simulink model "dobdesign"  (R2022b)
settings: Solver=FixedStepAuto  StartTime=0.0  StopTime=inf  FixedStep=0.02  RelTol=1e-3
values from neighbouring files (symbols this model uses):
  acri = atan(1/theta)    [transfer.m]
  Cfa = 15000    [transfer.m]
  D = 0    [transfer.m]
  Fz = (m*g)/4    (= 3801.375)    [transfer.m]
  J = 2392    [transfer.m]
  m = 1550    [transfer.m]
  mu = 1    [transfer.m]
  V = 30    [transfer.m]
libraries: cstblocks x4, simulink x2, simulink_extras x1, fuzblock x1, slpidlib x1, vehdynlibviscommon x1
settings Model: Creator=clkgo  LastModifiedBy=clkgo
settings SolverCC: AlgebraicLoopSolver=TrustRegion
settings DebuggingCC: UnconnectedInputMsg=warning  UnconnectedOutputMsg=warning  UnconnectedLineMsg=warning  SFMachineParentedDataDiag=warning
settings ModelReferenceCC: EnableRefExpFcnMdlSchedulingChecks=on
settings RTWCC: DLArmComputeVersion=19.05

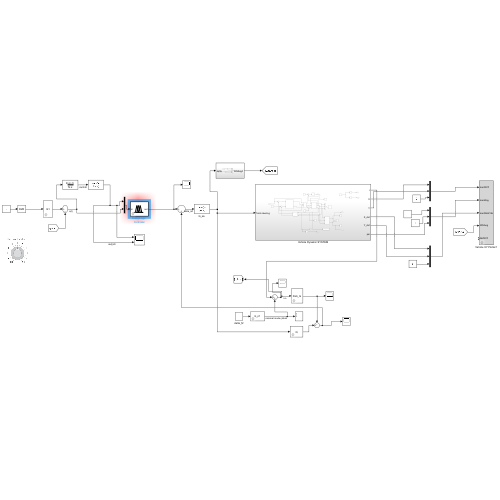
[thumbnail: Simulink's stored preview of the top-level diagram]
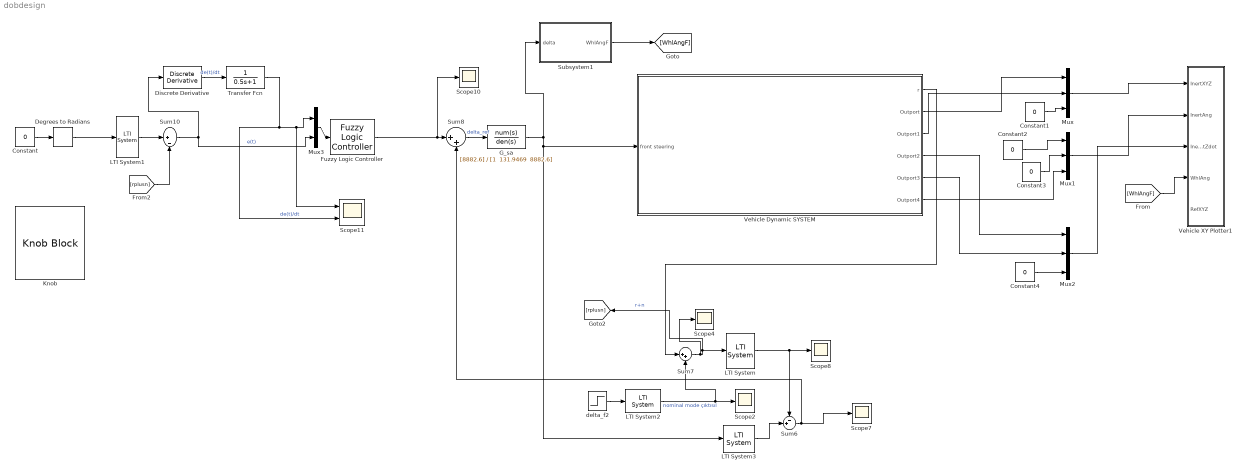
== system dobdesign ==
  Constant{,1..4} (5 alike) : Constant  Value=0
  Degrees to Radians : simulink_extras/Transformations/Degrees to Radians
  Discrete Derivative : simulink/Discrete/Discrete Derivative  gainval=1.0  ICPrevScaledInput=0.0  OutMin=[]  OutMax=[]  OutDataType=fixdt(1, 16)  OutScaling=2^-10  DoSatur=off
  Fuzzy Logic Controller : fuzblock/Fuzzy Logic  Controller  FIS=dobfuzzy14  OutputSampleNumber=101  DataType=double  FuzzifiedInputs=off  RuleFiringStrengths=off  RuleOutputs=off  AggregatedOutputs=off  SimulateUsing=Interpreted execution  OutOfRangeInputValueMessage=warning  NoRuleFiredMessage=warning  EmptyOutputFuzzySetMessage=warning
  "G_sa " : TransferFcn  Numerator=[8882.6]  Denominator="[1  131.9469  8882.6]"
  Knob : KnobBlock  ScaleMin=-10  ScaleMax=10
  LTI System : cstblocks/LTI System  sys=Dob_G  IC=[]
  LTI System1 : cstblocks/LTI System  sys=G1  IC=[]
  LTI System2 : cstblocks/LTI System  sys=G_n1  IC=[]
  LTI System3 : cstblocks/LTI System  sys=Q  IC=[]
  Mux : Mux  Inputs=3
  Mux1 : Mux  Inputs=3
  Mux2 : Mux  Inputs=3
  Mux3 : Mux  Inputs=2
  Scope{2,4,7..8,10} (5 alike) : Scope
  Scope11 : Scope  NumInputPorts=2
  Subsystem1 : Subsystem
  Sum10 : Sum  Inputs=|+-
  Sum6 : Sum  Inputs=-+|
  Sum7 : Sum  Inputs=|++
  Sum8 : Sum  Inputs=|++
  Transfer Fcn : TransferFcn  Denominator=[0.5 1]
  Vehicle Dynamic SYSTEM : Subsystem
  Vehicle XY Plotter1 : Subsystem  mask(Vehicle XY Plotter){extRef=on, extStats=off, extTireF=off, a=2, b=2, w=2, figBorder=10, bufferSize=1024, velNorm=5, tireFNorm=1000, pltDT=0.2}
      mask prompts: extRef "Plot path reference, extRef"; extStats "Display speed, RPM and Gear"; extTireF "Display tire forces"; a "Distance to front axle from CG, a [m]:"; b "Distance to rear axle from CG, b [m]:"; w "Track width, w [m]:"; figBorder "Distance to figure borders, figBorder [m]:"; bufferSize "Path buffer sampe size, bufferSize []:"; velNorm "Velocity vector scaling, velNorm [m*s/m]:"; tireFNorm "Tire force vector scaling, tireFNorm [m/N]:"; pltDT "Plot update rate, pltDT [s]:"
      mask help:
      | This block will display a MATLAB figure which indicates the vehicle path, current position and heading velocity.
      | An optional path reference is also provided.
      mask init:
      | block = gcb;
      | if autoblkschecksimstopped(block)
      |     ParamNames = {'extRef';'extStats';'extTireF';'extTireF'};
      |     PortNames = {'RefXYZ';'Stats';'TireFx';'TireFy'};
      |     for idx=1:length(PortNames)
      |         InportOption  = {'built-in/Ground', [PortNames{idx}, ' Ground'];...
      |             'built-in/Inport',PortNames{idx}};
      |         if ~strcmp(get_param(block,ParamNames{idx}),'on')
      |             NewBlkHdl = autoblksreplaceblock(block, InportOption, 1);
      |             set_param(NewBlkHdl, 'ShowName', 'off');
      |         else
      |             autoblksreplaceblock(block, InportOption, 2);
      |         end
      |     end
      |     InportNames = {'InertXYZ';'InertAng';'InertXdotYdotZdot';'WhlAng';'RefXYZ';'Stats';'TireFx';'TireFy'};
      |     FoundNames = get_param(find_system(block, 'LookUnderMasks', 'all', 'SearchDepth', 1, 'FollowLinks', 'on', 'BlockType', 'Inport'), 'Name');
      |     [~,PortI] = intersect(InportNames, FoundNames);
      |     PortI = sort(PortI);
      |     for idx = 1:length(PortI)
      |         set_param([block, '/', InportNames{PortI(idx)}], 'Port', num2str(idx));
      |     end
      | end
      mask TypeOptions a: Vehicle XY Plotter/a
      mask TypeOptions b: Vehicle XY Plotter/b
      mask TypeOptions w: Vehicle XY Plotter/w
      mask TypeOptions figBorder: Vehicle XY Plotter/figBorder
      mask TypeOptions bufferSize: Vehicle XY Plotter/bufferSize
      mask TypeOptions velNorm: Vehicle XY Plotter/velNorm
      mask TypeOptions tireFNorm: Vehicle XY Plotter/tireFNorm
      mask DialogControl Container3 Prompt: Plot and Display Options
  delta_f2 : Step  Time=0.1  After=0  SampleTime=0
  wires:
  Vehicle Dynamic SYSTEM/1(r) -> Sum7/1
  LTI System/1 -> Sum6/1, Scope8/1
  LTI System2/1 -> Scope2/1, Sum7/2  "nominal mode çıktısıl"
  "G_sa "/1 -> LTI System3/1, Vehicle Dynamic SYSTEM/1(front steering), Subsystem1/1(delta)
  Sum7/1 -> Scope4/1, LTI System/1, [rplusn]  "r+n"
  LTI System3/1 -> Sum6/2
  Sum6/1 -> Sum8/2, Scope7/1
  Sum8/1 -> "G_sa "/1  "delta_ref"
  delta_f2/1 -> LTI System2/1
  [rplusn] -> Sum10/2
  LTI System1/1 -> Sum10/1
  Degrees to Radians/1 -> LTI System1/1
  Sum10/1 -> Mux3/2, Discrete Derivative/1  "e(t)"
  Mux3/1 -> Fuzzy Logic Controller/1
  Discrete Derivative/1 -> Transfer Fcn/1  "de(t)/dt"
  Transfer Fcn/1 -> Scope11/2, Scope11/1, Mux3/1  "de(t)/dt"
  Fuzzy Logic Controller/1 -> Scope10/1, Sum8/1
  Constant/1 -> Degrees to Radians/1
  Subsystem1/1(WhlAngF) -> [WhlAngF]
  Vehicle Dynamic SYSTEM/2(Outport) -> Mux/1
  Vehicle Dynamic SYSTEM/3(Outport1) -> Mux/2
  Constant1/1 -> Mux/3
  Mux/1 -> Vehicle XY Plotter1/1(InertXYZ)
  Constant2/1 -> Mux1/1
  Constant3/1 -> Mux1/2
  Vehicle Dynamic SYSTEM/6(Outport4) -> Mux1/3
  Mux1/1 -> Vehicle XY Plotter1/2(InertAng)
  Vehicle Dynamic SYSTEM/4(Outport2) -> Mux2/1
  Vehicle Dynamic SYSTEM/5(Outport3) -> Mux2/2
  Constant4/1 -> Mux2/3
  Mux2/1 -> Vehicle XY Plotter1/3(InertXdotYdotZdot)
  [WhlAngF] -> Vehicle XY Plotter1/4(WhlAng)

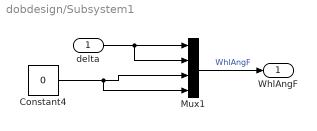
== system dobdesign/Subsystem1 ==
  delta : Inport
  Constant4 : Constant  Value=0
  Mux1 : Mux
  WhlAngF : Outport
  wires:
  delta/1 -> Mux1/2, Mux1/1
  Mux1/1 -> WhlAngF/1  "WhlAngF"
  Constant4/1 -> Mux1/4, Mux1/3

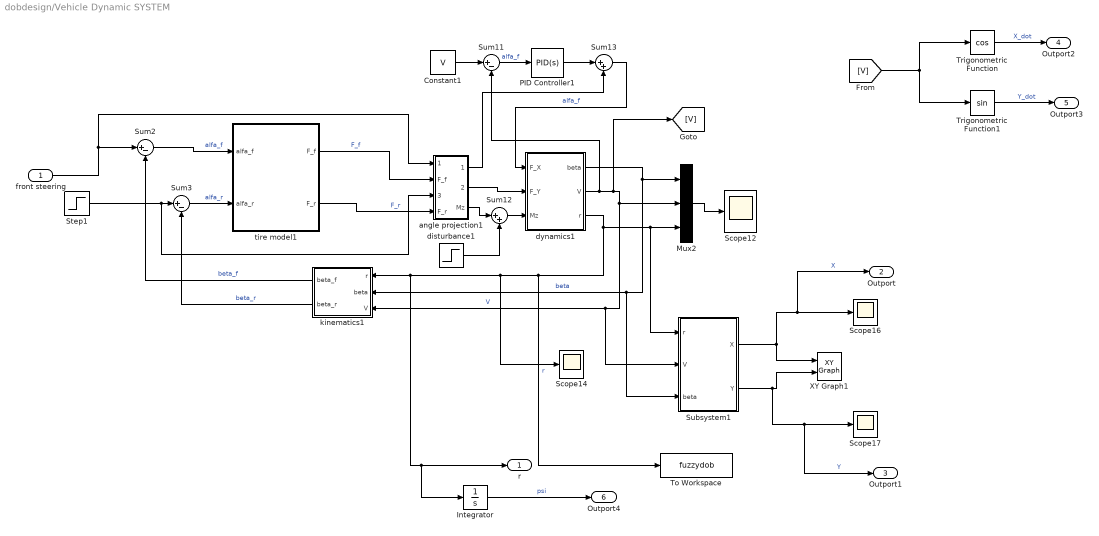
== system dobdesign/Vehicle Dynamic SYSTEM ==
  front steering : Inport
  Constant1 : Constant  Value=V
  Integrator : Integrator
  Mux2 : Mux  Inputs=3
  PID Controller1 : slpidlib/PID Controller  Controller=PID  Form=Parallel  TimeDomain=Continuous-time  UseExternalTs=off  SampleTime=-1  IntegratorMethod=Forward Euler  FilterMethod=Forward Euler  ControllerParametersSource=internal  P=60000  I=1000  D=0  UseFilter=on  N=100  TunerSelectOption=Transfer Function Based (PID Tuner App)  InitialConditionSource=internal  InitialConditionForIntegrator=0  InitialConditionForFilter=0  DifferentiatorICPrevScaledInput=0  ExternalReset=none  TrackingMode=off  Kt=1  LimitOutput=off  SatLimitsSource=internal  UpperSaturationLimit=inf  LowerSaturationLimit=-inf  LinearizeAsGain=on  AntiWindupMode=none  Kb=1  POutMin=[]  POutMax=[]  IOutMin=[]  IOutMax=[]  DOutMin=[]  DOutMax=[]  NOutMin=[]  NOutMax=[]  SumOutMin=[]  SumOutMax=[]  SaturationOutMin=[]  SaturationOutMax=[]  PParamMin=[]  PParamMax=[]  IParamMin=[]  IParamMax=[]  DParamMin=[]  DParamMax=[]  NParamMin=[]  NParamMax=[]  KbParamMin=[]  KbParamMax=[]  KtParamMin=[]  KtParamMax=[]  KbOutMin=[]  KbOutMax=[]  KtOutMin=[]  KtOutMax=[]  IntegratorOutMin=[]  IntegratorOutMax=[]  FilterOutMin=[]  FilterOutMax=[]  SumI1OutMin=[]  SumI1OutMax=[]  SumI2OutMin=[]  SumI2OutMax=[]  SumI3OutMin=[]  SumI3OutMax=[]  SumI4OutMin=[]  SumI4OutMax=[]  SumDOutMin=[]  SumDOutMax=[]  DifferentiatorOutMin=[]  DifferentiatorOutMax=[]  FilterDiffOutCoefMin=[]  FilterDiffOutCoefMax=[]  ReciprocalOutMin=[]  ReciprocalOutMax=[]  SumDenOutMin=[]  SumDenOutMax=[]  SumNumOutMin=[]  SumNumOutMax=[]  DivideOutMin=[]  DivideOutMax=[]  UdiffTsProdOutMin=[]  UdiffTsProdOutMax=[]  NTsProdOutMin=[]  NTsProdOutMax=[]  UintegralTsProdOutMin=[]  UintegralTsProdOutMax=[]  UngainTsProdOutMin=[]  UngainTsProdOutMax=[]  IntegratorContinuousStateAttributes=''  IntegratorStateMustResolveToSignalObject=off  IntegratorRTWStateStorageClass=Auto  FilterContinuousStateAttributes=''  FilterStateMustResolveToSignalObject=off  FilterRTWStateStorageClass=Auto  ParallelPVariant=InternalParameters  IdealPVariant=Disabled  IVariant=InternalParameters  DVariant=InternalParameters  IntegratorVariant=Continuous  SatVariant=Disabled  AWVariant=Passthrough  PCopyVariant=Disabled  TRVariant=Disabled  FdbkBlocksVariant=Forward  IdealPFdbkVariant=Disabled  SatFdbkVariant=Disabled  DerivativeFilterVariant=ContFilter  NVariant=InternalParameters  NCopyVariant=Disabled  FilterICVariant=InternalICsFilter  IntegratorICVariant=InternalICs  ExternalResetVariant=Disabled  TRSumVariant=Passthrough  SumFdbkVariant=Disabled  SumVariant=Sum_PID  TsampFilterVariant=InternalTs  TsampNgainVariant=Passthrough  TsampIntegralVariant=Passthrough  ExternalSaturationOutDataTypeStr=Inherit: Same as second input
  Scope{12,14,16..17} (4 alike) : Scope
  Step1 : Step  Time=0.1  After=0  SampleTime=0
  Subsystem1 : Subsystem
  Sum11 : Sum  Inputs=|+-
  Sum12 : Sum  Inputs=|++
  Sum13 : Sum  Inputs=|++
  Sum2 : Sum  Inputs=|+-
  Sum3 : Sum  Inputs=|+-
  To Workspace : ToWorkspace  VariableName=fuzzydob  SaveFormat=Timeseries  SampleTime=-1
  Trigonometric Function : Trigonometry  Operator=cos
  Trigonometric Function1 : Trigonometry
  XY Graph1 : simulink/Sinks/XY Graph  xmin=0  xmax=500  ymin=0  ymax=50  st=-1
  angle projection1 : Subsystem
  disturbance1 : Step  Time=2  After=1000  SampleTime=0
  dynamics1 : Subsystem
  kinematics1 : Subsystem
  tire model1 : Subsystem
  r : Outport
  Outport : Outport  Port=2
  Outport1 : Outport  Port=3
  Outport2 : Outport  Port=4
  Outport3 : Outport  Port=5
  Outport4 : Outport  Port=6
  wires:
  kinematics1/1(beta_f) -> Sum2/2  "beta_f"
  dynamics1/3(r) -> To Workspace/1, Scope14/1, Integrator/1, r/1, kinematics1/1(r), Subsystem1/1(r), Mux2/3  "r"
  Sum2/1 -> tire model1/1(alfa_f)  "alfa_f"
  dynamics1/2(V) -> [V], Subsystem1/2(V), kinematics1/3(V), Mux2/2, Sum11/2  "V"
  dynamics1/1(beta) -> Subsystem1/3(beta), kinematics1/2(beta), Mux2/1  "beta"
  kinematics1/2(beta_r) -> Sum3/2  "beta_r"
  Subsystem1/2(Y) -> Outport1/1, Scope17/1, XY Graph1/2  "Y"
  disturbance1/1 -> Sum12/2
  Sum3/1 -> tire model1/2(alfa_r)  "alfa_r"
  PID Controller1/1 -> Sum13/1
  Step1/1 -> angle projection1/3(In3), Sum3/1
  Constant1/1 -> Sum11/1
  tire model1/1(F_f) -> angle projection1/2(F_f)  "F_f"
  angle projection1/3(Mz) -> Sum12/1
  tire model1/2(F_r) -> angle projection1/4(F_r)  "F_r"
  angle projection1/2(F_Y) -> dynamics1/2(F_Y)
  angle projection1/1(F_X) -> Sum13/2
  Mux2/1 -> Scope12/1
  Sum11/1 -> PID Controller1/1  "alfa_f"
  Sum12/1 -> dynamics1/3(Mz)
  front steering/1 -> angle projection1/1(In1), Sum2/1
  Subsystem1/1(X) -> XY Graph1/1, Outport/1, Scope16/1  "X"
  Sum13/1 -> dynamics1/1(F_X)  "alfa_f"
  [V] -> Trigonometric Function/1, Trigonometric Function1/1
  Trigonometric Function/1 -> Outport2/1  "X_dot"
  Trigonometric Function1/1 -> Outport3/1  "Y_dot"
  Integrator/1 -> Outport4/1  "psi"

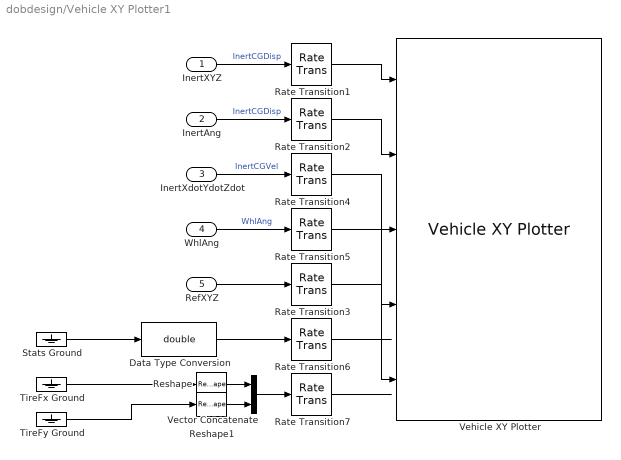
== system dobdesign/Vehicle XY Plotter1 ==
  InertXYZ : Inport
  InertAng : Inport  Port=2
  InertXdotYdotZdot : Inport  Port=3
  WhlAng : Inport  Port=4
  RefXYZ : Inport  Port=5
  Data Type Conversion : DataTypeConversion  OutDataTypeStr=double  SaturateOnIntegerOverflow=off  RndMeth=Floor
  Rate Transition{1..7} (7 alike) : RateTransition  Deterministic=off  OutPortSampleTime=pltDT
  Reshape : Reshape  OutputDimensionality=Row vector (2-D)
  Reshape1 : Reshape  OutputDimensionality=Row vector (2-D)
  Stats Ground : Ground
  TireFx Ground : Ground
  TireFy Ground : Ground
  Vector Concatenate : Concatenate  Mode=Multidimensional array
  Vehicle XY Plotter : vehdynlibviscommon/Vehicle XY Plotter  w=w  a=a  b=b  figBorder=figBorder  bufferSize=bufferSize  extStats=off  extTireF=off
  wires:
  Vector Concatenate/1 -> Rate Transition7/1
  Reshape1/1 -> Vector Concatenate/2
  Reshape/1 -> Vector Concatenate/1
  RefXYZ/1 -> Rate Transition3/1
  Rate Transition7/1 -> ?
  Data Type Conversion/1 -> Rate Transition6/1
  Rate Transition6/1 -> ?
  Rate Transition5/1 -> Vehicle XY Plotter/4
  Rate Transition4/1 -> Vehicle XY Plotter/3
  Rate Transition2/1 -> Vehicle XY Plotter/2
  Rate Transition1/1 -> Vehicle XY Plotter/1
  Rate Transition3/1 -> Vehicle XY Plotter/5
  WhlAng/1 -> Rate Transition5/1  "WhlAng"
  InertXYZ/1 -> Rate Transition1/1  "InertCGDisp"
  InertXdotYdotZdot/1 -> Rate Transition4/1  "InertCGVel"
  InertAng/1 -> Rate Transition2/1  "InertCGDisp"
  Stats Ground/1 -> Data Type Conversion/1
  TireFx Ground/1 -> Reshape/1
  TireFy Ground/1 -> Reshape1/1

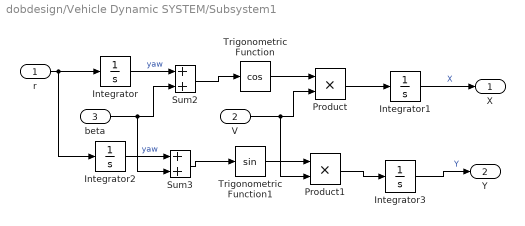
== system dobdesign/Vehicle Dynamic SYSTEM/Subsystem1 ==
  r : Inport
  V : Inport  Port=2
  beta : Inport  Port=3
  Integrator : Integrator
  Integrator1 : Integrator  UpperSaturationLimit=80  LowerSaturationLimit=0
  Integrator2 : Integrator
  Integrator3 : Integrator  UpperSaturationLimit=80  LowerSaturationLimit=0
  Product : Product
  Product1 : Product
  Sum2 : Sum
  Sum3 : Sum
  Trigonometric Function : Trigonometry  Operator=cos
  Trigonometric Function1 : Trigonometry
  X : Outport
  Y : Outport  Port=2
  wires:
  Integrator/1 -> Sum2/1  "yaw"
  V/1 -> Product1/2, Product/2
  Sum2/1 -> Trigonometric Function/1
  Product1/1 -> Integrator3/1
  Trigonometric Function/1 -> Product/1
  Trigonometric Function1/1 -> Product1/1
  Sum3/1 -> Trigonometric Function1/1
  Product/1 -> Integrator1/1
  Integrator2/1 -> Sum3/1  "yaw"
  Integrator3/1 -> Y/1  "Y"
  Integrator1/1 -> X/1  "X"
  beta/1 -> Sum3/2, Sum2/2
  r/1 -> Integrator2/1, Integrator/1

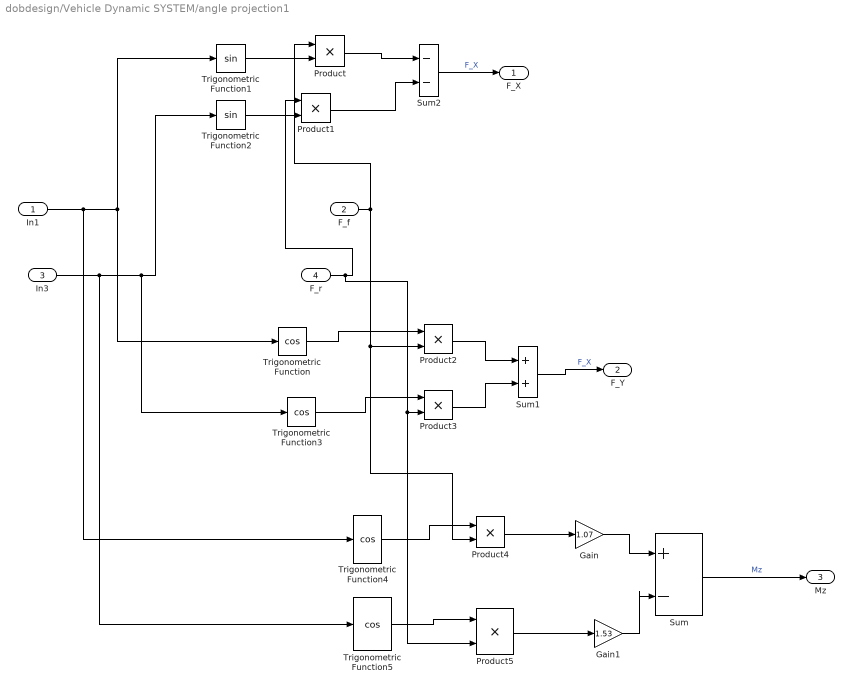
== system dobdesign/Vehicle Dynamic SYSTEM/angle projection1 ==
  In1 : Inport
  F_f : Inport  Port=2
  In3 : Inport  Port=3
  F_r : Inport  Port=4
  Gain : Gain  Gain=1.07
  Gain1 : Gain  Gain=1.53
  Product{,1..5} (6 alike) : Product
  Sum : Sum  Inputs=+-
  Sum1 : Sum
  Sum2 : Sum  Inputs=--
  Trigonometric Function{,3..5} (4 alike) : Trigonometry  Operator=cos
  Trigonometric Function1 : Trigonometry
  Trigonometric Function2 : Trigonometry
  F_X : Outport
  F_Y : Outport  Port=2
  Mz : Outport  Port=3
  wires:
  Trigonometric Function2/1 -> Product1/2
  Sum2/1 -> F_X/1  "F_X"
  Product1/1 -> Sum2/2
  F_f/1 -> Product/1, Product2/2, Product4/2
  Trigonometric Function1/1 -> Product/2
  F_r/1 -> Product5/2, Product3/2, Product1/1
  In3/1 -> Trigonometric Function5/1, Trigonometric Function3/1, Trigonometric Function2/1
  Product/1 -> Sum2/1
  In1/1 -> Trigonometric Function4/1, Trigonometric Function1/1, Trigonometric Function/1
  Trigonometric Function/1 -> Product2/1
  Trigonometric Function3/1 -> Product3/1
  Product2/1 -> Sum1/1
  Product3/1 -> Sum1/2
  Sum1/1 -> F_Y/1  "F_X"
  Trigonometric Function4/1 -> Product4/1
  Trigonometric Function5/1 -> Product5/1
  Product4/1 -> Gain/1
  Product5/1 -> Gain1/1
  Gain/1 -> Sum/1
  Gain1/1 -> Sum/2
  Sum/1 -> Mz/1  "Mz"

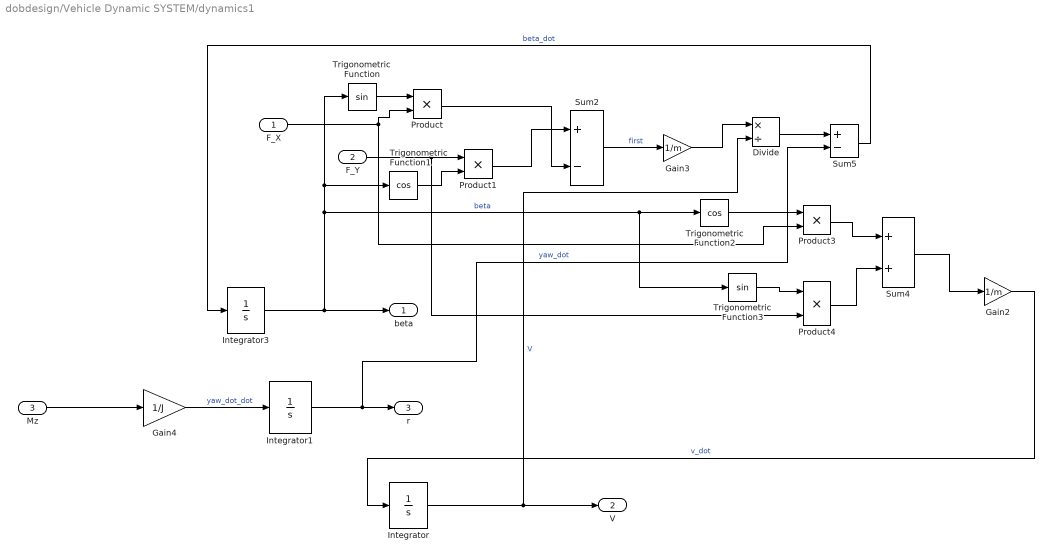
== system dobdesign/Vehicle Dynamic SYSTEM/dynamics1 ==
  F_X : Inport
  F_Y : Inport  Port=2
  Mz : Inport  Port=3
  Divide : Product  Inputs=*/
  Gain2 : Gain  Gain=1/m
  Gain3 : Gain  Gain=1/m
  Gain4 : Gain  Gain=1/J
  Integrator : Integrator  InitialCondition=V
  Integrator1 : Integrator
  Integrator3 : Integrator
  Product{,1,3..4} (4 alike) : Product
  Sum2 : Sum  Inputs=+-
  Sum4 : Sum
  Sum5 : Sum  Inputs=+-
  Trigonometric Function : Trigonometry
  Trigonometric Function1 : Trigonometry  Operator=cos
  Trigonometric Function2 : Trigonometry  Operator=cos
  Trigonometric Function3 : Trigonometry
  beta : Outport
  V : Outport  Port=2
  r : Outport  Port=3
  wires:
  Trigonometric Function1/1 -> Product1/2
  Gain3/1 -> Divide/1
  Integrator1/1 -> r/1, Sum5/2  "yaw_dot"
  F_Y/1 -> Product4/2, Product1/1
  Gain4/1 -> Integrator1/1  "yaw_dot_dot"
  Mz/1 -> Gain4/1
  Sum2/1 -> Gain3/1  "first"
  Divide/1 -> Sum5/1
  F_X/1 -> Product/2, Product3/2
  Gain2/1 -> Integrator/1  "v_dot"
  Sum5/1 -> Integrator3/1  "beta_dot"
  Product3/1 -> Sum4/1
  Sum4/1 -> Gain2/1
  Product4/1 -> Sum4/2
  Trigonometric Function2/1 -> Product3/1
  Integrator/1 -> V/1, Divide/2  "V"
  Trigonometric Function3/1 -> Product4/1
  Integrator3/1 -> beta/1, Trigonometric Function3/1, Trigonometric Function2/1, Trigonometric Function1/1, Trigonometric Function/1  "beta"
  Trigonometric Function/1 -> Product/1
  Product1/1 -> Sum2/1
  Product/1 -> Sum2/2

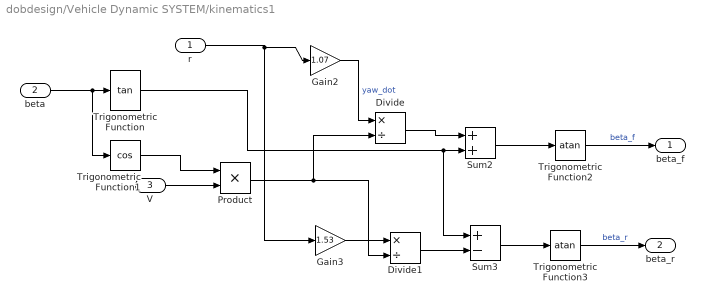
== system dobdesign/Vehicle Dynamic SYSTEM/kinematics1 ==
  r : Inport
  beta : Inport  Port=2
  V : Inport  Port=3
  Divide : Product  Inputs=*/
  Divide1 : Product  Inputs=*/
  Gain2 : Gain  Gain=1.07
  Gain3 : Gain  Gain=1.53
  Product : Product
  Sum2 : Sum
  Sum3 : Sum  Inputs=+-
  Trigonometric Function : Trigonometry  Operator=tan
  Trigonometric Function1 : Trigonometry  Operator=cos
  Trigonometric Function2 : Trigonometry  Operator=atan
  Trigonometric Function3 : Trigonometry  Operator=atan
  beta_f : Outport
  beta_r : Outport  Port=2
  wires:
  Product/1 -> Divide1/2, Divide/2
  Gain2/1 -> Divide/1  "yaw_dot"
  Sum3/1 -> Trigonometric Function3/1
  Trigonometric Function/1 -> Sum2/2, Sum3/1
  beta/1 -> Trigonometric Function1/1, Trigonometric Function/1
  Divide/1 -> Sum2/1
  Gain3/1 -> Divide1/1
  Trigonometric Function1/1 -> Product/1
  Sum2/1 -> Trigonometric Function2/1
  Divide1/1 -> Sum3/2
  r/1 -> Gain3/1, Gain2/1
  Trigonometric Function3/1 -> beta_r/1  "beta_r"
  Trigonometric Function2/1 -> beta_f/1  "beta_f"
  V/1 -> Product/2

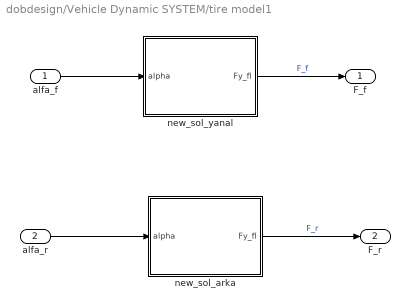
== system dobdesign/Vehicle Dynamic SYSTEM/tire model1 ==
  alfa_f : Inport
  alfa_r : Inport  Port=2
  new_sol_arka : MATLAB Function  TreatAsAtomicUnit=on
  new_sol_yanal : MATLAB Function  TreatAsAtomicUnit=on
  F_f : Outport
  F_r : Outport  Port=2
  wires:
  new_sol_arka/1(Fy_fl) -> F_r/1  "F_r"
  alfa_f/1 -> new_sol_yanal/1(alpha)
  new_sol_yanal/1(Fy_fl) -> F_f/1  "F_f"
  alfa_r/1 -> new_sol_arka/1(alpha)

== matlab function dobdesign/Vehicle Dynamic SYSTEM/tire model1/new_sol_arka ==
  data: alpha input; Fy_fl output; Fz parameter; mu parameter; Cfa parameter; acri parameter
function Fy_fl = fcn(alpha,Fz, mu, Cfa, acri)
if abs(alpha)<= acri
    Fy_fl= Cfa*(tan(alpha))- (((Cfa^2)/(3*mu*Fz))*tan(alpha)*abs(tan(alpha)))+ ((Cfa^3)/(27*(mu^2)*(Fz^2)))*(tan(alpha)^3);
    
else 
    Fy_fl= mu*Fz*sign(alpha);
end

== matlab function dobdesign/Vehicle Dynamic SYSTEM/tire model1/new_sol_yanal ==
  data: alpha input; Fy_fl output; Fz parameter; mu parameter; Cfa parameter; acri parameter
function Fy_fl = fcn(alpha,Fz, mu, Cfa, acri)
if abs(alpha)<= acri
    Fy_fl= Cfa*(tan(alpha))- (((Cfa^2)/(3*mu*Fz))*tan(alpha)*abs(tan(alpha)))+ ((Cfa^3)/(27*(mu^2)*(Fz^2)))*(tan(alpha)^3);
    
else 
    Fy_fl= mu*Fz*sign(alpha);
end
